simulink model "lista2_przyklad"  (R2022b)
settings: Solver=FixedStepAuto  StartTime=0.0  StopTime=10.0  FixedStep=0.01  RelTol=1e-3
settings Model: Creator=mateu  LastModifiedBy=mateu

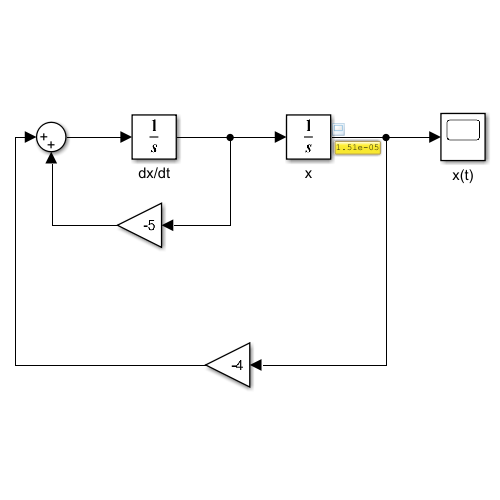
[thumbnail: Simulink's stored preview of the top-level diagram]
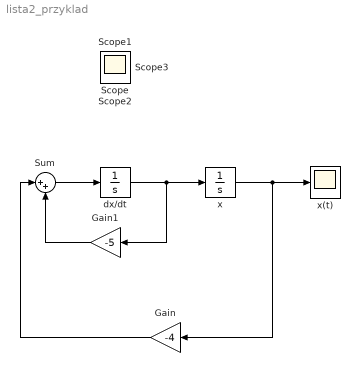
== system lista2_przyklad ==
  Gain : Gain  Gain=-4
  Gain1 : Gain  Gain=-5
  Sum : Sum  Inputs=|++
  dx/dt : Integrator  InitialCondition=1
  x : Integrator
  x(t) : Scope
  Scope{,1..3} (4 alike) : Scope
  wires:
  Gain/1 -> Sum/1
  Gain1/1 -> Sum/2
  Sum/1 -> dx/dt/1
  dx/dt/1 -> Gain1/1, x/1
  x/1 -> Gain/1, x(t)/1
